simulink library "NeuroModelerLibrary"  (Simulink 10.2)
settings: Solver=ode45  StartTime=0.0  StopTime=10.0  RelTol=1e-3
libraries: $bdroot x672, simulink x5, neural x2
(part 2 of 5)

== system NeuroModelerLibrary/Neuron Elements/IaF Compartment ==
  Synapses : Inport
  Resting Potential : Inport  Port=2
  Reset Signal : Inport  Port=3
  Constant1 : Constant  Value=V_reset
  Constant10 : Constant  Value=tau_m
  Constant12 : Constant  Value=I_const
  Gain3 : Gain  Gain=tau_m/Cm
  Inertial Link With Reset1 : $bdroot/Support/Inertial Link With Reset  SystemSampleTime=-1  VariantActivationTime=update diagram  Latency=0  AutoFrameSizeCalculation=off
  Sum1 : Sum
  Sum3 : Sum
  Out1 : Outport
  wires:
  Reset Signal/1 -> Inertial Link With Reset1/4
  Gain3/1 -> Sum3/1  "Input"
  Constant1/1 -> Inertial Link With Reset1/3
  Inertial Link With Reset1/1 -> Out1/1
  Sum3/1 -> Inertial Link With Reset1/1  "Value"
  Constant12/1 -> Sum1/2
  Sum1/1 -> Gain3/1
  Synapses/1 -> Sum1/1
  Constant10/1 -> Inertial Link With Reset1/2
  Resting Potential/1 -> Sum3/2

== system NeuroModelerLibrary/Neuron Elements/IaF LTZone ==
  Potential : Inport
  Constant2 : Constant
  Constant6 : Constant  Value=0
  S1 : Switch  Threshold=V_th  SaturateOnIntegerOverflow=on  InputSameDT=on
  Out : Outport
  Out Potential : Outport  Port=2
  wires:
  S1/1 -> Out/1
  Potential/1 -> S1/2, Out Potential/1
  Constant6/1 -> S1/3
  Constant2/1 -> S1/1

== system NeuroModelerLibrary/Neuron Elements/Ion System ==
  Synapse : Inport
  Channel : Inport  Port=2
  Rm : Inport  Port=3
  Cm : Inport  Port=4
  Feedback : Inport  Port=5
  RFm : Inport  Port=6
  Divide : Product  Inputs=*/
  Divide1 : Product  Inputs=*/
  F1 : Fcn  Expr=-u
  F4 : Fcn  Expr=1/u
  Inertial Link : $bdroot/Support/Inertial Link  SystemSampleTime=-1  VariantActivationTime=update diagram  Latency=0  AutoFrameSizeCalculation=off
  P1 : Product  InputSameDT=on  RndMeth=Zero  SaturateOnIntegerOverflow=on  OutDataTypeStr=Inherit: Same as first input
  S2 : Switch  Criteria=u2 > Threshold  SaturateOnIntegerOverflow=on  InputSameDT=on
  Sum2 : Sum  InputSameDT=on  SaturateOnIntegerOverflow=on  OutDataTypeStr=Inherit: Same as first input
  Sum4 : Sum  Inputs=-+  InputSameDT=on  SaturateOnIntegerOverflow=on  OutDataTypeStr=Inherit: Same as first input
  Sum5 : Sum  InputSameDT=on  SaturateOnIntegerOverflow=on  OutDataTypeStr=Inherit: Same as first input
  Out : Outport  VectorParamsAs1DForOutWhenUnconnected=off
  wires:
  F1/1 -> Sum2/1
  Channel/1 -> Sum2/2
  Sum2/1 -> Sum4/2
  Feedback/1 -> F1/1, S2/2
  Rm/1 -> S2/3
  RFm/1 -> S2/1
  S2/1 -> F4/1
  Sum4/1 -> Inertial Link/1
  P1/1 -> Sum4/1
  Inertial Link/1 -> Out/1, P1/1
  Sum5/1 -> Divide/2
  Divide/1 -> Inertial Link/2
  Synapse/1 -> Divide1/1, Sum5/2
  F4/1 -> Divide1/2, Sum5/1
  Cm/1 -> Divide/1
  Divide1/1 -> P1/2

== system NeuroModelerLibrary/Neuron Elements/Ion System v0.1 ==
  Synapse : Inport
  Channel : Inport  Port=2
  Rm : Inport  Port=3
  Cm : Inport  Port=4
  Divide : Product  Inputs=**/  InputSameDT=on  RndMeth=Zero  OutDataTypeStr=Inherit: Same as first input
  F2 : Fcn  Expr=u
  F3 : Fcn  Expr=1/(1+abs(u))
  F4 : Fcn  Expr=1/u
  Inertial Link (H1) : Subsystem
  P1 : Product  InputSameDT=on  RndMeth=Zero  SaturateOnIntegerOverflow=on  OutDataTypeStr=Inherit: Same as first input
  Product : Product  InputSameDT=on  RndMeth=Zero  OutDataTypeStr=Inherit: Same as first input
  Sum1 : Sum  Inputs=-+  InputSameDT=on  SaturateOnIntegerOverflow=on  OutDataTypeStr=Inherit: Same as first input
  Sum4 : Sum  Inputs=-+  InputSameDT=on  SaturateOnIntegerOverflow=on  OutDataTypeStr=Inherit: Same as first input
  Sum5 : Sum  InputSameDT=on  SaturateOnIntegerOverflow=on  OutDataTypeStr=Inherit: Same as first input
  Out : Outport  VectorParamsAs1DForOutWhenUnconnected=off
  wires:
  Sum4/1 -> Inertial Link (H1)/1(In1)
  P1/1 -> Sum4/1
  Inertial Link (H1)/1(Out1) -> P1/1, Out/1, Sum1/2
  Sum5/1 -> Divide/3
  Divide/1 -> Inertial Link (H1)/2(In2)
  Synapse/1 -> Product/1, Sum5/2
  Channel/1 -> Sum4/2, Sum1/1
  Rm/1 -> F4/1, F2/1
  F4/1 -> Sum5/1
  Cm/1 -> Divide/1
  F2/1 -> Product/2
  Product/1 -> P1/2
  F3/1 -> Divide/2
  Sum1/1 -> F3/1

== system NeuroModelerLibrary/Neuron Elements/LTZone ==
  Potential : Inport
  E : Inport  Port=2
  C5 : Constant  Value=0
  FB : Gain  Gain=FB  OutDataTypeStr=Inherit: Same as input  ParamDataTypeStr=Inherit: Same as input
  Inputs : Gain  Gain=1/NM  OutDataTypeStr=Inherit: Same as input  ParamDataTypeStr=Inherit: Same as input
  Relay : Relay  OnSwitchValue=T  OffSwitchValue=0
  S2 : Switch  Threshold=1  SaturateOnIntegerOverflow=on  InputSameDT=on
  S3 : Switch  Threshold=1  SaturateOnIntegerOverflow=on  InputSameDT=on
  Transfer Fcn : TransferFcn  Denominator=[IT 1]
  Feedback : Outport  InitialOutput=0  VectorParamsAs1DForOutWhenUnconnected=off
  Visual : Outport  Port=2  InitialOutput=0  VectorParamsAs1DForOutWhenUnconnected=off
  Out : Outport  Port=3  InitialOutput=0  VectorParamsAs1DForOutWhenUnconnected=off
  wires:
  Transfer Fcn/1 -> S3/3, Relay/1
  S3/1 -> Visual/1
  Relay/1 -> S3/2, S2/2
  S2/1 -> FB/1, Out/1
  E/1 -> S2/1, S3/1
  C5/1 -> S2/3
  Potential/1 -> Inputs/1
  FB/1 -> Feedback/1
  Inputs/1 -> Transfer Fcn/1

== system NeuroModelerLibrary/Neuron Elements/LTZone v0.1 ==
  note: X1
  note: X2
  Sum : Inport
  E : Inport  Port=2
  C1 : Constant
  C2 : Constant  Value=1/Rc
  C3 : Constant  Value=1/RR
  C5 : Constant  Value=0
  F1 : Fcn  Expr=Cc/u
  Inertial Link (H1) : Subsystem
  Relay : Relay  OnSwitchValue=T  OffSwitchValue=0
  S1 : Switch  Threshold=1  SaturateOnIntegerOverflow=on  InputSameDT=on
  S2 : Switch  Threshold=1  SaturateOnIntegerOverflow=on  InputSameDT=on
  S3 : Switch  Threshold=1  SaturateOnIntegerOverflow=on  InputSameDT=on
  Sum2 : Sum  InputSameDT=on  SaturateOnIntegerOverflow=on  OutDataTypeStr=Inherit: Same as first input
  Transfer Fcn : TransferFcn  Denominator=[IT 1]
  Out : Outport  InitialOutput=0  VectorParamsAs1DForOutWhenUnconnected=off
  Membrane : Outport  Port=2  InitialOutput=0  VectorParamsAs1DForOutWhenUnconnected=off
  Visual : Outport  Port=3  InitialOutput=0  VectorParamsAs1DForOutWhenUnconnected=off
  wires:
  S3/1 -> Visual/1
  Relay/1 -> S3/2, S2/2, S1/2
  Transfer Fcn/1 -> Membrane/1, S3/3, Relay/1, Sum2/2
  S1/1 -> F1/1
  S2/1 -> Out/1, Sum2/1
  E/1 -> S3/1, S2/1
  C5/1 -> S2/3
  Sum/1 -> Transfer Fcn/1
  C3/1 -> S1/1
  C2/1 -> S1/3
  F1/1 -> Inertial Link (H1)/2(In2)
  Sum2/1 -> Inertial Link (H1)/1(In1)

== system NeuroModelerLibrary/Neuron Elements/LTZoneV2 ==
  Potential : Inport
  E : Inport  Port=2
  C1 : Constant  Value=inertia
  C5 : Constant  Value=0
  FB : Gain  Gain=FB  OutDataTypeStr=Inherit: Same as input  ParamDataTypeStr=Inherit: Same as input
  Inputs : Gain  Gain=1/NM  OutDataTypeStr=Inherit: Same as input  ParamDataTypeStr=Inherit: Same as input
  Relay : Relay  OnSwitchValue=T  OffSwitchValue=switchOff
  S2 : Switch  Threshold=1  SaturateOnIntegerOverflow=on  InputSameDT=on
  S3 : Switch  Threshold=1  SaturateOnIntegerOverflow=on  InputSameDT=on
  Switch : Switch  Threshold=1
  Transfer Fcn1 : TransferFcn  Denominator=[IT 1]
  Out : Outport  InitialOutput=0  VectorParamsAs1DForOutWhenUnconnected=off
  OutPotential : Outport  Port=2  InitialOutput=0  VectorParamsAs1DForOutWhenUnconnected=off
  Feedback : Outport  Port=3  InitialOutput=0  VectorParamsAs1DForOutWhenUnconnected=off
  Visual : Outport  Port=4  InitialOutput=0  VectorParamsAs1DForOutWhenUnconnected=off
  wires:
  Transfer Fcn1/1 -> Switch/1
  C1/1 -> Switch/2
  Inputs/1 -> Switch/3, Transfer Fcn1/1
  Switch/1 -> S3/3, OutPotential/1, Relay/1
  S3/1 -> Visual/1
  Relay/1 -> S3/2, S2/2
  S2/1 -> FB/1, Out/1
  E/1 -> S2/1, S3/1
  C5/1 -> S2/3
  Potential/1 -> Inputs/1
  FB/1 -> Feedback/1

== system NeuroModelerLibrary/Neuron Elements/Multistate Membrane ==
  Excitatory Synapse : Inport
  Excitatory input : Inport  Port=2
  Feedback : Inport  Port=3
  Arresting input : Inport  Port=4
  Arresting Synapse : Inport  Port=5
  Gain5 : Gain  Gain=0.5  OutDataTypeStr=Inherit: Same as input  ParamDataTypeStr=Inherit: Same as input
  Gain6 : Gain  Gain=0.5  OutDataTypeStr=Inherit: Same as input  ParamDataTypeStr=Inherit: Same as input
  Simple Membrane : $bdroot/Neuron Elements/Simple Membrane  ACm=1e-9  ARm=1e7  ECm=1e-9  ERm=1e7  ARFm=1e8  ERFm=1e8
  Simple Membrane1 : $bdroot/Neuron Elements/Simple Membrane  ACm=1e-9  ARm=1e7  ECm=1e-9  ERm=1e7  ARFm=1e8  ERFm=1e8
  Sum{1,3,8..11} (6 alike) : Sum  InputSameDT=on  SaturateOnIntegerOverflow=on  OutDataTypeStr=Inherit: Same as first input
  Out1 : Outport  VectorParamsAs1DForOutWhenUnconnected=off
  Out3 : Outport  Port=2  VectorParamsAs1DForOutWhenUnconnected=off
  wires:
  Arresting input/1 -> Sum9/1, Sum11/1
  Sum1/1 -> Gain5/1
  Sum3/1 -> Gain6/1
  Simple Membrane/2 -> Sum3/1, Sum11/2
  Simple Membrane/1 -> Sum1/1, Sum10/1
  Gain5/1 -> Out1/1
  Gain6/1 -> Out3/1
  Sum8/1 -> Simple Membrane/2
  Sum9/1 -> Simple Membrane/4
  Sum10/1 -> Simple Membrane1/2
  Sum11/1 -> Simple Membrane1/4
  Simple Membrane1/1 -> Sum9/2, Sum1/2
  Simple Membrane1/2 -> Sum8/1, Sum3/2
  Feedback/1 -> Simple Membrane/3, Simple Membrane1/3
  Excitatory Synapse/1 -> Simple Membrane1/1
  Arresting Synapse/1 -> Simple Membrane1/5
  Excitatory input/1 -> Sum8/2, Sum10/2

== system NeuroModelerLibrary/Neuron Elements/Neuro Membrane v0.1 ==
  Excitatory Synapse : Inport
  Excitatory Channel : Inport  Port=2
  Recharge : Inport  Port=3
  Arresting Channel : Inport  Port=4
  Arresting Synapse : Inport  Port=5
  ACm : Constant  Value=ACm
  ARm : Constant  Value=ARm
  ECm : Constant  Value=ECm
  ERm : Constant  Value=ERm
  Neuro Channel : $bdroot/Neuron Elements/Ion System v0.1  SystemSampleTime=-1  VariantActivationTime=update diagram  Latency=0  AutoFrameSizeCalculation=off
  Neuro Channel1 : $bdroot/Neuron Elements/Ion System v0.1  SystemSampleTime=-1  VariantActivationTime=update diagram  Latency=0  AutoFrameSizeCalculation=off
  Sum1 : Sum  Inputs=-+  InputSameDT=on  SaturateOnIntegerOverflow=on  OutDataTypeStr=Inherit: Same as first input
  Sum2 : Sum  Inputs=+-  InputSameDT=on  SaturateOnIntegerOverflow=on  OutDataTypeStr=Inherit: Same as first input
  Excitatory Out : Outport  VectorParamsAs1DForOutWhenUnconnected=off
  Arresting Out : Outport  Port=2  VectorParamsAs1DForOutWhenUnconnected=off
  wires:
  Recharge/1 -> Sum2/2, Sum1/1
  Arresting Channel/1 -> Sum2/1
  Sum2/1 -> Neuro Channel/2
  Sum1/1 -> Neuro Channel1/2
  Excitatory Channel/1 -> Sum1/2
  Arresting Synapse/1 -> Neuro Channel1/1
  Excitatory Synapse/1 -> Neuro Channel/1
  Neuro Channel/1 -> Arresting Out/1
  Neuro Channel1/1 -> Excitatory Out/1
  ERm/1 -> Neuro Channel1/3
  ECm/1 -> Neuro Channel1/4
  ARm/1 -> Neuro Channel/3
  ACm/1 -> Neuro Channel/4

== system NeuroModelerLibrary/Neuron Elements/Simple Membrane ==
  Excitatory Synapse : Inport
  Excitatory input : Inport  Port=2
  Feedback : Inport  Port=3
  Arresting input : Inport  Port=4
  Arresting Synapse : Inport  Port=5
  ACm : Constant  Value=ACm
  ARm : Constant  Value=ARm
  ARm1 : Constant  Value=ARFm
  ECm : Constant  Value=ECm
  ERm : Constant  Value=ERm
  ERm1 : Constant  Value=ERFm
  Ion System : $bdroot/Neuron Elements/Ion System
  Ion System1 : $bdroot/Neuron Elements/Ion System
  Excitatory Out : Outport  VectorParamsAs1DForOutWhenUnconnected=off
  Arresting Out : Outport  Port=2  VectorParamsAs1DForOutWhenUnconnected=off
  wires:
  Arresting input/1 -> Ion System/2
  Feedback/1 -> Ion System/5, Ion System1/5
  ARm1/1 -> Ion System/6
  Excitatory input/1 -> Ion System1/2
  Arresting Synapse/1 -> Ion System1/1
  Excitatory Synapse/1 -> Ion System/1
  ERm/1 -> Ion System1/3
  ECm/1 -> Ion System1/4
  ARm/1 -> Ion System/3
  ACm/1 -> Ion System/4
  Ion System/1 -> Arresting Out/1
  ERm1/1 -> Ion System1/6
  Ion System1/1 -> Excitatory Out/1

== system NeuroModelerLibrary/Neuron Elements/Synapse ==
  In1 : Inport
  Constant1 : Constant  Value=0
  Constant2 : Constant  Value=UseKsi
  Constant4 : Constant  Value=DecompositionTC
  Constant5 : Constant  Value=SecretionTC
  Fcn : Fcn  Expr=u*u*ksi
  Gain : Gain  Gain=4*ksi/gamma  SaturateOnIntegerOverflow=on  OutDataTypeStr=Inherit: Same as input  ParamDataTypeStr=Inherit: Same as input
  Gain1 : Gain  SaturateOnIntegerOverflow=on  OutDataTypeStr=Inherit: Same as input  ParamDataTypeStr=Inherit: Same as input
  Gain2 : Gain  Gain=1/gamma  SaturateOnIntegerOverflow=on  OutDataTypeStr=Inherit: Same as input  ParamDataTypeStr=Inherit: Same as input
  Inertial Link : $bdroot/Support/Inertial Link
  Sum : Sum  Inputs=+-  SaturateOnIntegerOverflow=on
  Switch1 : Switch
  Switch2 : Switch  Threshold=1
  Switch3 : Switch  Threshold=1
  Out1 : Outport  VectorParamsAs1DForOutWhenUnconnected=off
  wires:
  Fcn/1 -> Sum/2
  In1/1 -> Switch2/2, Gain1/1
  Sum/1 -> Gain/1
  Inertial Link/1 -> Gain2/1, Fcn/1, Sum/1
  Constant4/1 -> Switch2/3
  Constant5/1 -> Switch2/1
  Switch2/1 -> Inertial Link/2
  Constant1/1 -> Switch1/3
  Gain1/1 -> Inertial Link/1
  Switch1/1 -> Out1/1
  Gain/1 -> Switch3/1
  Switch3/1 -> Switch1/1, Switch1/2
  Constant2/1 -> Switch3/2
  Gain2/1 -> Switch3/3

== system NeuroModelerLibrary/Neuron Elements/Synapse Ion System v0.1 ==
  Synapse : Inport
  Channel : Inport  Port=2
  Rm : Inport  Port=3
  Cm : Inport  Port=4
  Divide : Product  Inputs=**/  InputSameDT=on  RndMeth=Zero  OutDataTypeStr=Inherit: Same as first input
  F2 : Fcn  Expr=u
  F3 : Fcn  Expr=1/(1+abs(u))
  F4 : Fcn  Expr=1/u
  Inertial Link (H1) : Subsystem
  P1 : Product  Inputs=3  InputSameDT=on  RndMeth=Zero  SaturateOnIntegerOverflow=on  OutDataTypeStr=Inherit: Same as first input
  Product : Product  InputSameDT=on  RndMeth=Zero  OutDataTypeStr=Inherit: Same as first input
  Sum1 : Sum  Inputs=-+  InputSameDT=on  SaturateOnIntegerOverflow=on  OutDataTypeStr=Inherit: Same as first input
  Sum4 : Sum  Inputs=-+  InputSameDT=on  SaturateOnIntegerOverflow=on  OutDataTypeStr=Inherit: Same as first input
  Sum5 : Sum  InputSameDT=on  SaturateOnIntegerOverflow=on  OutDataTypeStr=Inherit: Same as first input
  Out : Outport  VectorParamsAs1DForOutWhenUnconnected=off
  wires:
  Sum1/1 -> F3/1
  Product/1 -> P1/2
  F2/1 -> Product/2
  F4/1 -> Sum5/1
  Rm/1 -> F2/1, F4/1
  Channel/1 -> Sum1/1, Sum4/2
  Synapse/1 -> Sum5/2, Product/1, P1/3
  Divide/1 -> Inertial Link (H1)/2(In2)
  Sum5/1 -> Divide/3
  Inertial Link (H1)/1(Out1) -> Sum1/2, Out/1, P1/1
  P1/1 -> Sum4/1
  Sum4/1 -> Inertial Link (H1)/1(In1)
  F3/1 -> Divide/1
  Cm/1 -> Divide/2

== system NeuroModelerLibrary/Neuron Elements/Synapse Membrane v0.1 ==
  Excitatory Synapse : Inport
  Excitatory Channel : Inport  Port=2
  Recharge : Inport  Port=3
  Arresting Channel : Inport  Port=4
  Arresting Synapse : Inport  Port=5
  ACm : Constant  Value=ACm
  ARm : Constant  Value=ARm
  ECm : Constant  Value=ECm
  ERm : Constant  Value=ERm
  Sum1 : Sum  Inputs=-+  InputSameDT=on  SaturateOnIntegerOverflow=on  OutDataTypeStr=Inherit: Same as first input
  Sum2 : Sum  Inputs=+-  InputSameDT=on  SaturateOnIntegerOverflow=on  OutDataTypeStr=Inherit: Same as first input
  Synapse Channel : $bdroot/Neuron Elements/Synapse Ion System v0.1  SystemSampleTime=-1  VariantActivationTime=update diagram  Latency=0  AutoFrameSizeCalculation=off
  Synapse Channel1 : $bdroot/Neuron Elements/Synapse Ion System v0.1  SystemSampleTime=-1  VariantActivationTime=update diagram  Latency=0  AutoFrameSizeCalculation=off
  Excitatory Out : Outport  VectorParamsAs1DForOutWhenUnconnected=off
  Arresting Out : Outport  Port=2  VectorParamsAs1DForOutWhenUnconnected=off
  wires:
  ACm/1 -> Synapse Channel/4
  ARm/1 -> Synapse Channel/3
  ECm/1 -> Synapse Channel1/4
  ERm/1 -> Synapse Channel1/3
  Synapse Channel1/1 -> Excitatory Out/1
  Synapse Channel/1 -> Arresting Out/1
  Excitatory Synapse/1 -> Synapse Channel/1
  Arresting Synapse/1 -> Synapse Channel1/1
  Excitatory Channel/1 -> Sum1/2
  Sum1/1 -> Synapse Channel1/2
  Sum2/1 -> Synapse Channel/2
  Arresting Channel/1 -> Sum2/1
  Recharge/1 -> Sum1/1, Sum2/2

== system NeuroModelerLibrary/Neuron Elements/Synapse v0.1 ==
  In1 : Inport
  Constant1 : Constant  Value=0
  Constant4 : Constant  Value=DecompositionTC
  Constant5 : Constant  Value=SecretionTC
  Fcn : Fcn  Expr=u*u*ksi
  Fcn1 : Fcn  Expr=u/(u+ksi)
  Gain : Gain  Gain=gamma*4*ksi  SaturateOnIntegerOverflow=on  OutDataTypeStr=Inherit: Same as input  ParamDataTypeStr=Inherit: Same as input
  Gain1 : Gain  Gain=0.01  SaturateOnIntegerOverflow=on  OutDataTypeStr=Inherit: Same as input  ParamDataTypeStr=Inherit: Same as input
  Inertial Link (H1)1 : Subsystem
  Sum : Sum  Inputs=+-  InputSameDT=on  SaturateOnIntegerOverflow=on  OutDataTypeStr=Inherit: Same as first input
  Switch1 : Switch  SaturateOnIntegerOverflow=on  InputSameDT=on
  Switch2 : Switch  Threshold=1  SaturateOnIntegerOverflow=on  InputSameDT=on
  Out1 : Outport  VectorParamsAs1DForOutWhenUnconnected=off
  wires:
  Fcn/1 -> Sum/2
  In1/1 -> Switch2/2, Gain1/1
  Sum/1 -> Gain/1
  Inertial Link (H1)1/1(Out1) -> Fcn/1, Sum/1
  Constant4/1 -> Switch2/3
  Constant5/1 -> Switch2/1
  Switch2/1 -> Inertial Link (H1)1/2(In2)
  Gain/1 -> Switch1/2, Switch1/1
  Constant1/1 -> Switch1/3
  Gain1/1 -> Inertial Link (H1)1/1(In1)
  Switch1/1 -> Out1/1

== system NeuroModelerLibrary/Pacemaker Cells/Pacemaker1-1 Cell ==
  Stimulate1 : Inport
  Stimulate2 : Inport  Port=2
  Stimulate3 : Inport  Port=3
  Stimulate4 : Inport  Port=4
  Arresting1 : Inport  Port=5
  Arresting2 : Inport  Port=6
  Arresting3 : Inport  Port=7
  Arresting4 : Inport  Port=8
  C1 : Constant
  C2 : Constant
  C3 : Constant  Value=-0.99
  LTZone : $bdroot/Neuron Elements/LTZone  SystemSampleTime=-1  NM=1  FB=1.7  IT=0.005  T=0.001
  Simple Membrane{,1..3} (4 alike) : $bdroot/Neuron Elements/Simple Membrane  SystemSampleTime=-1  ACm=1e-9  ARm=1e7  ECm=1e-9  ERm=1e7  ARFm=1e8  ERFm=1e8
  Sum12 : Sum  InputSameDT=on  SaturateOnIntegerOverflow=on  OutDataTypeStr=Inherit: Same as first input
  Sum7 : Sum  InputSameDT=on  SaturateOnIntegerOverflow=on  OutDataTypeStr=Inherit: Same as first input
  Synapse{,1..7} (8 alike) : $bdroot/Neuron Elements/Synapse  SystemSampleTime=-1  SecretionTC=0.001  DecompositionTC=0.01  ksi=2  gamma=1e8
  Out : Outport  VectorParamsAs1DForOutWhenUnconnected=off
  Visual : Outport  Port=2  VectorParamsAs1DForOutWhenUnconnected=off
  Potential : Outport  Port=3  VectorParamsAs1DForOutWhenUnconnected=off
  wires:
  Synapse7/1 -> Simple Membrane/5
  Arresting4/1 -> Synapse7/1
  Synapse6/1 -> Simple Membrane1/5
  Arresting3/1 -> Synapse6/1
  Synapse5/1 -> Simple Membrane2/5
  Arresting2/1 -> Synapse5/1
  Stimulate4/1 -> Synapse/1
  Synapse/1 -> Simple Membrane/1
  Stimulate3/1 -> Synapse1/1
  Synapse1/1 -> Simple Membrane1/1
  Stimulate2/1 -> Synapse2/1
  Synapse2/1 -> Simple Membrane2/1
  Synapse3/1 -> Simple Membrane3/1
  C2/1 -> Simple Membrane3/2
  C3/1 -> Simple Membrane3/4
  Synapse4/1 -> Simple Membrane3/5
  Simple Membrane3/2 -> Simple Membrane2/4
  Simple Membrane3/1 -> Simple Membrane2/2
  Simple Membrane2/2 -> Simple Membrane1/4
  Simple Membrane2/1 -> Simple Membrane1/2
  LTZone/2 -> Visual/1
  LTZone/3 -> Out/1
  C1/1 -> LTZone/2
  Stimulate1/1 -> Synapse3/1
  Arresting1/1 -> Synapse4/1
  Simple Membrane1/1 -> Sum12/1, Simple Membrane/2
  Simple Membrane1/2 -> Sum12/2, Simple Membrane/4
  Sum7/1 -> Potential/1, LTZone/1
  LTZone/1 -> Simple Membrane/3
  Simple Membrane/1 -> Sum7/1
  Simple Membrane/2 -> Sum7/2

== system NeuroModelerLibrary/Pacemaker Cells/Pacemaker1-2 Cell ==
  Stimulate1 : Inport
  Stimulate2 : Inport  Port=2
  Stimulate3 : Inport  Port=3
  Stimulate4 : Inport  Port=4
  Arresting1 : Inport  Port=5
  Arresting2 : Inport  Port=6
  Arresting3 : Inport  Port=7
  Arresting4 : Inport  Port=8
  C1 : Constant
  C2 : Constant
  C3 : Constant  Value=-0.99
  LTZone : $bdroot/Neuron Elements/LTZone  NM=1  FB=1.7  IT=0.005  T=0.001
  Simple Membrane{,1..3} (4 alike) : $bdroot/Neuron Elements/Simple Membrane  ACm=1e-9  ARm=1e7  ECm=1e-9  ERm=1e7  ARFm=1e8  ERFm=1e8
  Sum12 : Sum  InputSameDT=on  SaturateOnIntegerOverflow=on  OutDataTypeStr=Inherit: Same as first input
  Sum7 : Sum  InputSameDT=on  SaturateOnIntegerOverflow=on  OutDataTypeStr=Inherit: Same as first input
  Synapse{,1..7} (8 alike) : $bdroot/Neuron Elements/Synapse  SecretionTC=0.001  DecompositionTC=0.01  UseKsi=on  ksi=2  gamma=1e8
  Out : Outport  VectorParamsAs1DForOutWhenUnconnected=off
  Visual : Outport  Port=2  VectorParamsAs1DForOutWhenUnconnected=off
  Potential : Outport  Port=3  VectorParamsAs1DForOutWhenUnconnected=off
  wires:
  Simple Membrane/2 -> Sum7/2
  Simple Membrane/1 -> Sum7/1
  LTZone/1 -> Simple Membrane/3, Simple Membrane1/3
  Sum7/1 -> LTZone/1, Potential/1
  Simple Membrane1/2 -> Simple Membrane/4, Sum12/2
  Simple Membrane1/1 -> Simple Membrane/2, Sum12/1
  Arresting1/1 -> Synapse4/1
  Stimulate1/1 -> Synapse3/1
  C1/1 -> LTZone/2
  LTZone/3 -> Out/1
  LTZone/2 -> Visual/1
  Simple Membrane2/1 -> Simple Membrane1/2
  Simple Membrane2/2 -> Simple Membrane1/4
  Simple Membrane3/1 -> Simple Membrane2/2
  Simple Membrane3/2 -> Simple Membrane2/4
  Synapse4/1 -> Simple Membrane3/5
  C3/1 -> Simple Membrane3/4
  C2/1 -> Simple Membrane3/2
  Synapse3/1 -> Simple Membrane3/1
  Synapse2/1 -> Simple Membrane2/1
  Stimulate2/1 -> Synapse2/1
  Synapse1/1 -> Simple Membrane1/1
  Stimulate3/1 -> Synapse1/1
  Synapse/1 -> Simple Membrane/1
  Stimulate4/1 -> Synapse/1
  Arresting2/1 -> Synapse5/1
  Synapse5/1 -> Simple Membrane2/5
  Arresting3/1 -> Synapse6/1
  Synapse6/1 -> Simple Membrane1/5
  Arresting4/1 -> Synapse7/1
  Synapse7/1 -> Simple Membrane/5

== system NeuroModelerLibrary/Pacemaker Cells/Pacemaker1-3 Cell ==
  Stimulate1 : Inport
  Stimulate2 : Inport  Port=2
  Stimulate3 : Inport  Port=3
  Stimulate4 : Inport  Port=4
  Arresting1 : Inport  Port=5
  Arresting2 : Inport  Port=6
  Arresting3 : Inport  Port=7
  Arresting4 : Inport  Port=8
  C1 : Constant
  C2 : Constant
  C3 : Constant  Value=-0.99
  LTZone : $bdroot/Neuron Elements/LTZone  SystemSampleTime=-1  NM=1  FB=1.7  IT=0.005  T=0.001
  Simple Membrane{,1..3} (4 alike) : $bdroot/Neuron Elements/Simple Membrane  SystemSampleTime=-1  ACm=1e-9  ARm=1e7  ECm=1e-9  ERm=1e7  ARFm=1e8  ERFm=1e8
  Sum12 : Sum  InputSameDT=on  SaturateOnIntegerOverflow=on  OutDataTypeStr=Inherit: Same as first input
  Sum7 : Sum  InputSameDT=on  SaturateOnIntegerOverflow=on  OutDataTypeStr=Inherit: Same as first input
  Synapse{,1..7} (8 alike) : $bdroot/Neuron Elements/Synapse  SystemSampleTime=-1  SecretionTC=0.001  DecompositionTC=0.01  ksi=2  gamma=1e8
  Out : Outport  VectorParamsAs1DForOutWhenUnconnected=off
  Visual : Outport  Port=2  VectorParamsAs1DForOutWhenUnconnected=off
  Potential : Outport  Port=3  VectorParamsAs1DForOutWhenUnconnected=off
  wires:
  Synapse7/1 -> Simple Membrane/5
  Arresting4/1 -> Synapse7/1
  Synapse6/1 -> Simple Membrane1/5
  Arresting3/1 -> Synapse6/1
  Synapse5/1 -> Simple Membrane2/5
  Arresting2/1 -> Synapse5/1
  Stimulate4/1 -> Synapse/1
  Synapse/1 -> Simple Membrane/1
  Stimulate3/1 -> Synapse1/1
  Synapse1/1 -> Simple Membrane1/1
  Stimulate2/1 -> Synapse2/1
  Synapse2/1 -> Simple Membrane2/1
  Synapse3/1 -> Simple Membrane3/1
  C2/1 -> Simple Membrane3/2
  C3/1 -> Simple Membrane3/4
  Synapse4/1 -> Simple Membrane3/5
  Simple Membrane3/2 -> Simple Membrane2/4
  Simple Membrane3/1 -> Simple Membrane2/2
  Simple Membrane2/2 -> Simple Membrane1/4
  Simple Membrane2/1 -> Simple Membrane1/2
  LTZone/2 -> Visual/1
  LTZone/3 -> Out/1
  C1/1 -> LTZone/2
  Stimulate1/1 -> Synapse3/1
  Arresting1/1 -> Synapse4/1
  Simple Membrane1/1 -> Sum12/1, Simple Membrane/2
  Simple Membrane1/2 -> Sum12/2, Simple Membrane/4
  Sum7/1 -> Potential/1, LTZone/1
  LTZone/1 -> Simple Membrane/3, Simple Membrane1/3, Simple Membrane2/3
  Simple Membrane/1 -> Sum7/1
  Simple Membrane/2 -> Sum7/2

== system NeuroModelerLibrary/Pacemaker Cells/Pacemaker1-4 Cell ==
  Stimulate1 : Inport
  Stimulate2 : Inport  Port=2
  Stimulate3 : Inport  Port=3
  Stimulate4 : Inport  Port=4
  Arresting1 : Inport  Port=5
  Arresting2 : Inport  Port=6
  Arresting3 : Inport  Port=7
  Arresting4 : Inport  Port=8
  C1 : Constant
  C2 : Constant
  C3 : Constant  Value=-0.99
  LTZone : $bdroot/Neuron Elements/LTZone  NM=1  FB=1.7  IT=0.005  T=0.001
  Simple Membrane{,1..3} (4 alike) : $bdroot/Neuron Elements/Simple Membrane  ACm=1e-9  ARm=1e7  ECm=1e-9  ERm=1e7  ARFm=1e8  ERFm=1e8
  Sum12 : Sum  InputSameDT=on  SaturateOnIntegerOverflow=on  OutDataTypeStr=Inherit: Same as first input
  Sum7 : Sum  InputSameDT=on  SaturateOnIntegerOverflow=on  OutDataTypeStr=Inherit: Same as first input
  Synapse{,1..7} (8 alike) : $bdroot/Neuron Elements/Synapse  SecretionTC=0.001  DecompositionTC=0.01  UseKsi=on  ksi=2  gamma=1e8
  Out : Outport  VectorParamsAs1DForOutWhenUnconnected=off
  Visual : Outport  Port=2  VectorParamsAs1DForOutWhenUnconnected=off
  Potential : Outport  Port=3  VectorParamsAs1DForOutWhenUnconnected=off
  wires:
  Synapse7/1 -> Simple Membrane/5
  Arresting4/1 -> Synapse7/1
  Synapse6/1 -> Simple Membrane1/5
  Arresting3/1 -> Synapse6/1
  Synapse5/1 -> Simple Membrane2/5
  Arresting2/1 -> Synapse5/1
  Stimulate4/1 -> Synapse/1
  Synapse/1 -> Simple Membrane/1
  Stimulate3/1 -> Synapse1/1
  Synapse1/1 -> Simple Membrane1/1
  Stimulate2/1 -> Synapse2/1
  Synapse2/1 -> Simple Membrane2/1
  Synapse3/1 -> Simple Membrane3/1
  C2/1 -> Simple Membrane3/2
  C3/1 -> Simple Membrane3/4
  Synapse4/1 -> Simple Membrane3/5
  Simple Membrane3/2 -> Simple Membrane2/4
  Simple Membrane3/1 -> Simple Membrane2/2
  Simple Membrane2/2 -> Simple Membrane1/4
  Simple Membrane2/1 -> Simple Membrane1/2
  LTZone/2 -> Visual/1
  LTZone/3 -> Out/1
  C1/1 -> LTZone/2
  Stimulate1/1 -> Synapse3/1
  Arresting1/1 -> Synapse4/1
  Simple Membrane1/1 -> Sum12/1, Simple Membrane/2
  Simple Membrane1/2 -> Sum12/2, Simple Membrane/4
  Sum7/1 -> Potential/1, LTZone/1
  LTZone/1 -> Simple Membrane/3, Simple Membrane1/3, Simple Membrane2/3, Simple Membrane3/3
  Simple Membrane/1 -> Sum7/1
  Simple Membrane/2 -> Sum7/2

== system NeuroModelerLibrary/Pacemaker Cells/Pacemaker2 Cell ==
  Stimulate1 : Inport
  Stimulate2 : Inport  Port=2
  Stimulate3 : Inport  Port=3
  Stimulate4 : Inport  Port=4
  Arresting1 : Inport  Port=5
  Arresting2 : Inport  Port=6
  Arresting3 : Inport  Port=7
  Arresting4 : Inport  Port=8
  C1 : Constant
  C2 : Constant
  C3 : Constant  Value=-0.99
  C4 : Constant
  C5 : Constant  Value=-1
  LTZone : $bdroot/Neuron Elements/LTZone  SystemSampleTime=-1  NM=2  FB=1.2  IT=0.005  T=0.001
  Simple Membrane{,1..4} (5 alike) : $bdroot/Neuron Elements/Simple Membrane  SystemSampleTime=-1  ACm=1e-9  ARm=1e7  ECm=1e-9  ERm=1e7  ARFm=1e8  ERFm=1e8
  Sum1 : Sum  InputSameDT=on  SaturateOnIntegerOverflow=on  OutDataTypeStr=Inherit: Same as first input
  Sum12 : Sum  InputSameDT=on  SaturateOnIntegerOverflow=on  OutDataTypeStr=Inherit: Same as first input
  Sum7 : Sum  Inputs=++++  InputSameDT=on  SaturateOnIntegerOverflow=on  OutDataTypeStr=Inherit: Same as first input
  Synapse{,1..7} (8 alike) : $bdroot/Neuron Elements/Synapse  SystemSampleTime=-1  SecretionTC=0.001  DecompositionTC=0.01  ksi=2  gamma=1e8
  Out : Outport  VectorParamsAs1DForOutWhenUnconnected=off
  Visual : Outport  Port=2  VectorParamsAs1DForOutWhenUnconnected=off
  Potential : Outport  Port=3  VectorParamsAs1DForOutWhenUnconnected=off
  wires:
  C5/1 -> Simple Membrane4/4
  C4/1 -> Simple Membrane4/2
  Simple Membrane/1 -> Sum7/2
  Simple Membrane/2 -> Sum7/3
  Simple Membrane4/2 -> Sum1/2
  Simple Membrane4/1 -> Sum1/1
  LTZone/1 -> Simple Membrane/3, Simple Membrane4/3
  Sum7/1 -> Potential/1, LTZone/1
  Simple Membrane1/2 -> Sum12/2, Simple Membrane/4
  Simple Membrane1/1 -> Sum12/1, Simple Membrane/2
  Arresting1/1 -> Synapse4/1
  Stimulate1/1 -> Synapse3/1
  C1/1 -> LTZone/2
  LTZone/3 -> Out/1
  LTZone/2 -> Visual/1
  Simple Membrane2/1 -> Simple Membrane1/2
  Simple Membrane2/2 -> Simple Membrane1/4
  Simple Membrane3/1 -> Simple Membrane2/2
  Simple Membrane3/2 -> Simple Membrane2/4
  Synapse4/1 -> Simple Membrane3/5
  C3/1 -> Simple Membrane3/4
  C2/1 -> Simple Membrane3/2
  Synapse3/1 -> Simple Membrane3/1
  Synapse2/1 -> Simple Membrane2/1
  Stimulate2/1 -> Synapse2/1
  Synapse1/1 -> Simple Membrane1/1
  Stimulate3/1 -> Synapse1/1
  Synapse/1 -> Simple Membrane/1
  Stimulate4/1 -> Synapse/1
  Arresting2/1 -> Synapse5/1
  Synapse5/1 -> Simple Membrane2/5
  Arresting3/1 -> Synapse6/1
  Synapse6/1 -> Simple Membrane1/5
  Arresting4/1 -> Synapse7/1
  Synapse7/1 -> Simple Membrane/5
  Sum1/1 -> Sum7/1

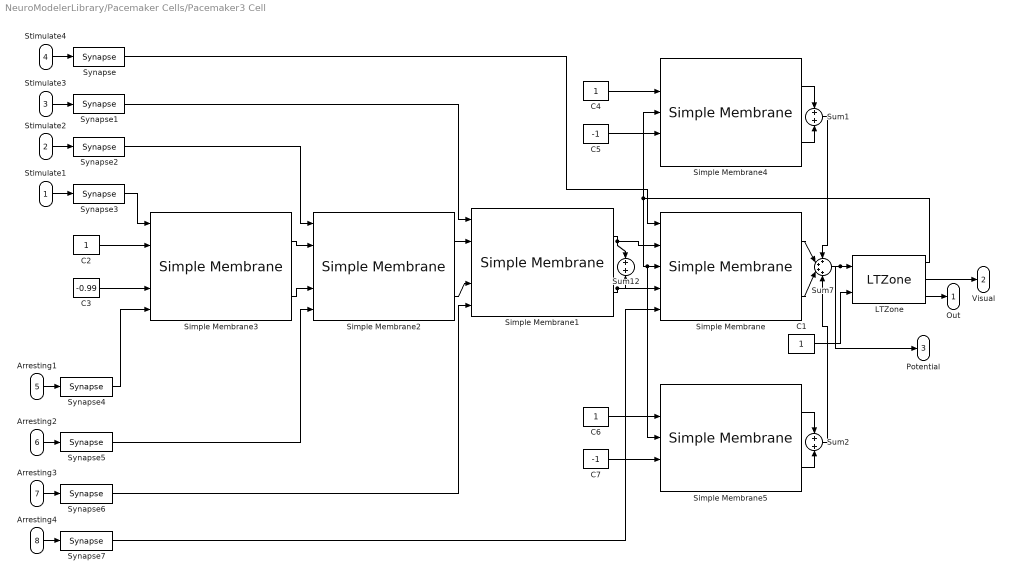
== system NeuroModelerLibrary/Pacemaker Cells/Pacemaker3 Cell ==
  Stimulate1 : Inport
  Stimulate2 : Inport  Port=2
  Stimulate3 : Inport  Port=3
  Stimulate4 : Inport  Port=4
  Arresting1 : Inport  Port=5
  Arresting2 : Inport  Port=6
  Arresting3 : Inport  Port=7
  Arresting4 : Inport  Port=8
  C{1..2,4,6} (4 alike) : Constant
  C3 : Constant  Value=-0.99
  C5 : Constant  Value=-1
  C7 : Constant  Value=-1
  LTZone : $bdroot/Neuron Elements/LTZone  SystemSampleTime=-1  NM=3  FB=1  IT=0.005  T=0.001
  Simple Membrane{,1..5} (6 alike) : $bdroot/Neuron Elements/Simple Membrane  SystemSampleTime=-1  ACm=1e-9  ARm=1e7  ECm=1e-9  ERm=1e7  ARFm=1e8  ERFm=1e8
  Sum1 : Sum  InputSameDT=on  SaturateOnIntegerOverflow=on  OutDataTypeStr=Inherit: Same as first input
  Sum12 : Sum  InputSameDT=on  SaturateOnIntegerOverflow=on  OutDataTypeStr=Inherit: Same as first input
  Sum2 : Sum  InputSameDT=on  SaturateOnIntegerOverflow=on  OutDataTypeStr=Inherit: Same as first input
  Sum7 : Sum  Inputs=++++  InputSameDT=on  SaturateOnIntegerOverflow=on  OutDataTypeStr=Inherit: Same as first input
  Synapse{,1..7} (8 alike) : $bdroot/Neuron Elements/Synapse  SystemSampleTime=-1  SecretionTC=0.001  DecompositionTC=0.01  ksi=2  gamma=1e8
  Out : Outport  VectorParamsAs1DForOutWhenUnconnected=off
  Visual : Outport  Port=2  VectorParamsAs1DForOutWhenUnconnected=off
  Potential : Outport  Port=3  VectorParamsAs1DForOutWhenUnconnected=off
  wires:
  Sum2/1 -> Sum7/4
  Simple Membrane5/1 -> Sum2/1
  Simple Membrane5/2 -> Sum2/2
  C6/1 -> Simple Membrane5/2
  C7/1 -> Simple Membrane5/4
  Synapse7/1 -> Simple Membrane/5
  Arresting4/1 -> Synapse7/1
  Synapse6/1 -> Simple Membrane1/5
  Arresting3/1 -> Synapse6/1
  Synapse5/1 -> Simple Membrane2/5
  Arresting2/1 -> Synapse5/1
  Stimulate4/1 -> Synapse/1
  Synapse/1 -> Simple Membrane/1
  Stimulate3/1 -> Synapse1/1
  Synapse1/1 -> Simple Membrane1/1
  Stimulate2/1 -> Synapse2/1
  Synapse2/1 -> Simple Membrane2/1
  Synapse3/1 -> Simple Membrane3/1
  C2/1 -> Simple Membrane3/2
  C3/1 -> Simple Membrane3/4
  Synapse4/1 -> Simple Membrane3/5
  Simple Membrane3/2 -> Simple Membrane2/4
  Simple Membrane3/1 -> Simple Membrane2/2
  Simple Membrane2/2 -> Simple Membrane1/4
  Simple Membrane2/1 -> Simple Membrane1/2
  LTZone/2 -> Visual/1
  LTZone/3 -> Out/1
  C1/1 -> LTZone/2
  Stimulate1/1 -> Synapse3/1
  Arresting1/1 -> Synapse4/1
  Simple Membrane1/1 -> Sum12/1, Simple Membrane/2
  Simple Membrane1/2 -> Sum12/2, Simple Membrane/4
  Sum7/1 -> Potential/1, LTZone/1
  LTZone/1 -> Simple Membrane/3, Simple Membrane5/3, Simple Membrane4/3
  Simple Membrane4/1 -> Sum1/1
  Simple Membrane4/2 -> Sum1/2
  Sum1/1 -> Sum7/1
  Simple Membrane/2 -> Sum7/3
  Simple Membrane/1 -> Sum7/2
  C4/1 -> Simple Membrane4/2
  C5/1 -> Simple Membrane4/4

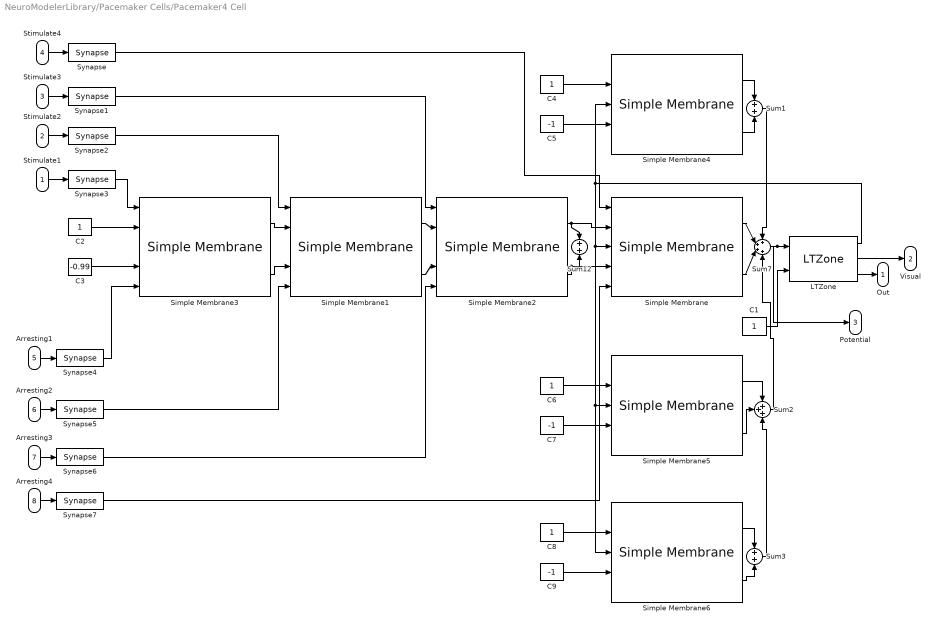
== system NeuroModelerLibrary/Pacemaker Cells/Pacemaker4 Cell ==
  Stimulate1 : Inport
  Stimulate2 : Inport  Port=2
  Stimulate3 : Inport  Port=3
  Stimulate4 : Inport  Port=4
  Arresting1 : Inport  Port=5
  Arresting2 : Inport  Port=6
  Arresting3 : Inport  Port=7
  Arresting4 : Inport  Port=8
  C{1..2,4,6,8} (5 alike) : Constant
  C3 : Constant  Value=-0.99
  C5 : Constant  Value=-1
  C7 : Constant  Value=-1
  C9 : Constant  Value=-1
  LTZone : $bdroot/Neuron Elements/LTZone  SystemSampleTime=-1  NM=4  FB=0.9  IT=0.005  T=0.001
  Simple Membrane{,1..6} (7 alike) : $bdroot/Neuron Elements/Simple Membrane  SystemSampleTime=-1  ACm=1e-9  ARm=1e7  ECm=1e-9  ERm=1e7  ARFm=1e8  ERFm=1e8
  Sum1 : Sum  InputSameDT=on  SaturateOnIntegerOverflow=on  OutDataTypeStr=Inherit: Same as first input
  Sum12 : Sum  InputSameDT=on  SaturateOnIntegerOverflow=on  OutDataTypeStr=Inherit: Same as first input
  Sum2 : Sum  Inputs=+++  InputSameDT=on  SaturateOnIntegerOverflow=on  OutDataTypeStr=Inherit: Same as first input
  Sum3 : Sum  InputSameDT=on  SaturateOnIntegerOverflow=on  OutDataTypeStr=Inherit: Same as first input
  Sum7 : Sum  Inputs=++++  InputSameDT=on  SaturateOnIntegerOverflow=on  OutDataTypeStr=Inherit: Same as first input
  Synapse{,1..7} (8 alike) : $bdroot/Neuron Elements/Synapse  SystemSampleTime=-1  SecretionTC=0.001  DecompositionTC=0.01  ksi=2  gamma=1e8
  Out : Outport  VectorParamsAs1DForOutWhenUnconnected=off
  Visual : Outport  Port=2  VectorParamsAs1DForOutWhenUnconnected=off
  Potential : Outport  Port=3  VectorParamsAs1DForOutWhenUnconnected=off
  wires:
  Sum3/1 -> Sum2/3
  Simple Membrane5/2 -> Sum2/2
  C9/1 -> Simple Membrane6/4
  C8/1 -> Simple Membrane6/2
  Simple Membrane6/2 -> Sum3/2
  Simple Membrane6/1 -> Sum3/1
  C5/1 -> Simple Membrane4/4
  C4/1 -> Simple Membrane4/2
  Simple Membrane/1 -> Sum7/2
  Simple Membrane/2 -> Sum7/3
  Sum1/1 -> Sum7/1
  Simple Membrane4/2 -> Sum1/2
  Simple Membrane4/1 -> Sum1/1
  LTZone/1 -> Simple Membrane5/3, Simple Membrane6/3, Simple Membrane/3, Simple Membrane4/3
  Sum7/1 -> Potential/1, LTZone/1
  Simple Membrane2/2 -> Sum12/2, Simple Membrane/4
  Simple Membrane2/1 -> Sum12/1, Simple Membrane/2
  Arresting1/1 -> Synapse4/1
  Stimulate1/1 -> Synapse3/1
  C1/1 -> LTZone/2
  LTZone/3 -> Out/1
  LTZone/2 -> Visual/1
  Simple Membrane1/1 -> Simple Membrane2/2
  Simple Membrane1/2 -> Simple Membrane2/4
  Simple Membrane3/1 -> Simple Membrane1/2
  Simple Membrane3/2 -> Simple Membrane1/4
  Synapse4/1 -> Simple Membrane3/5
  C3/1 -> Simple Membrane3/4
  C2/1 -> Simple Membrane3/2
  Synapse3/1 -> Simple Membrane3/1
  Synapse2/1 -> Simple Membrane1/1
  Stimulate2/1 -> Synapse2/1
  Synapse1/1 -> Simple Membrane2/1
  Stimulate3/1 -> Synapse1/1
  Synapse/1 -> Simple Membrane/1
  Stimulate4/1 -> Synapse/1
  Arresting2/1 -> Synapse5/1
  Synapse5/1 -> Simple Membrane1/5
  Arresting3/1 -> Synapse6/1
  Synapse6/1 -> Simple Membrane2/5
  Arresting4/1 -> Synapse7/1
  Synapse7/1 -> Simple Membrane/5
  C7/1 -> Simple Membrane5/4
  C6/1 -> Simple Membrane5/2
  Simple Membrane5/1 -> Sum2/1
  Sum2/1 -> Sum7/4

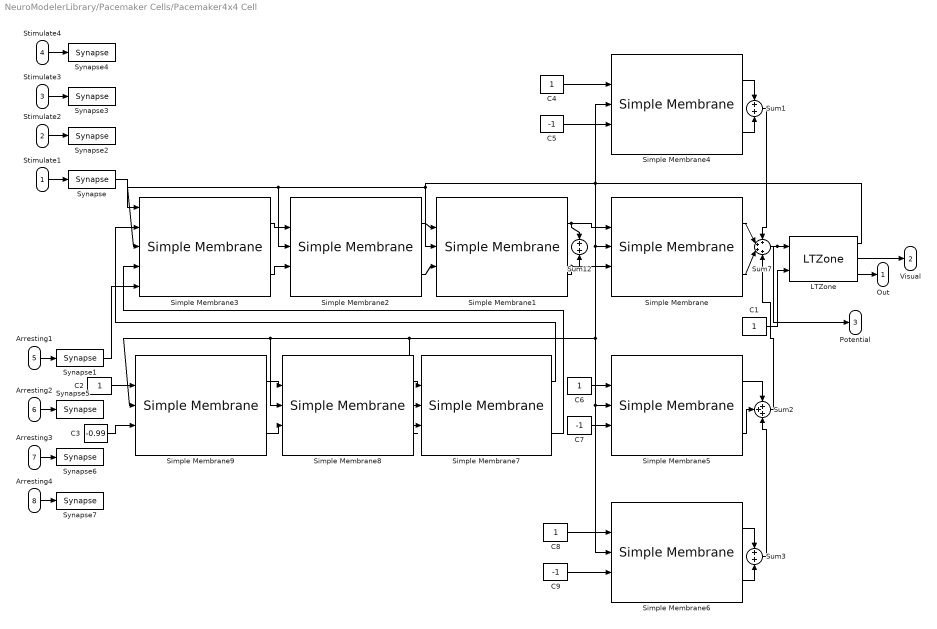
== system NeuroModelerLibrary/Pacemaker Cells/Pacemaker4x4 Cell ==
  Stimulate1 : Inport
  Stimulate2 : Inport  Port=2
  Stimulate3 : Inport  Port=3
  Stimulate4 : Inport  Port=4
  Arresting1 : Inport  Port=5
  Arresting2 : Inport  Port=6
  Arresting3 : Inport  Port=7
  Arresting4 : Inport  Port=8
  C{1..2,4,6,8} (5 alike) : Constant
  C3 : Constant  Value=-0.99
  C5 : Constant  Value=-1
  C7 : Constant  Value=-1
  C9 : Constant  Value=-1
  LTZone : $bdroot/LTZone  SystemSampleTime=-1  NM=4  FB=sqrt(4)  IT=0.005  T=0.001
  Simple Membrane{,1..9} (10 alike) : $bdroot/Simple Membrane  SystemSampleTime=-1  ACm=1e-9  ARm=1e7  ECm=1e-9  ERm=1e7  ARFm=1e8  ERFm=1e8
  Sum1 : Sum  InputSameDT=on  SaturateOnIntegerOverflow=on  OutDataTypeStr=Inherit: Same as first input
  Sum12 : Sum  InputSameDT=on  SaturateOnIntegerOverflow=on  OutDataTypeStr=Inherit: Same as first input
  Sum2 : Sum  Inputs=+++  InputSameDT=on  SaturateOnIntegerOverflow=on  OutDataTypeStr=Inherit: Same as first input
  Sum3 : Sum  InputSameDT=on  SaturateOnIntegerOverflow=on  OutDataTypeStr=Inherit: Same as first input
  Sum7 : Sum  Inputs=++++  InputSameDT=on  SaturateOnIntegerOverflow=on  OutDataTypeStr=Inherit: Same as first input
  Synapse{,1..7} (8 alike) : $bdroot/Synapse  SystemSampleTime=-1  SecretionTC=0.001  DecompositionTC=0.01  ksi=1  gamma=1e8
  Out : Outport  VectorParamsAs1DForOutWhenUnconnected=off
  Visual : Outport  Port=2  VectorParamsAs1DForOutWhenUnconnected=off
  Potential : Outport  Port=3  VectorParamsAs1DForOutWhenUnconnected=off
  wires:
  C3/1 -> Simple Membrane9/4
  C2/1 -> Simple Membrane9/2
  Simple Membrane9/2 -> Simple Membrane8/4
  Simple Membrane9/1 -> Simple Membrane8/2
  Simple Membrane8/2 -> Simple Membrane7/4
  Simple Membrane8/1 -> Simple Membrane7/2
  Simple Membrane7/1 -> Simple Membrane3/2
  Simple Membrane7/2 -> Simple Membrane3/4
  C9/1 -> Simple Membrane6/4
  C8/1 -> Simple Membrane6/2
  C7/1 -> Simple Membrane5/4
  C6/1 -> Simple Membrane5/2
  C5/1 -> Simple Membrane4/4
  C4/1 -> Simple Membrane4/2
  Sum3/1 -> Sum2/3
  Simple Membrane5/2 -> Sum2/2
  Simple Membrane6/2 -> Sum3/2
  Simple Membrane6/1 -> Sum3/1
  Simple Membrane/1 -> Sum7/2
  Simple Membrane/2 -> Sum7/3
  Sum1/1 -> Sum7/1
  Simple Membrane4/2 -> Sum1/2
  Simple Membrane4/1 -> Sum1/1
  LTZone/1 -> Simple Membrane3/3, Simple Membrane2/3, Simple Membrane1/3, Simple Membrane4/3, Simple Membrane9/3, Simple Membrane8/3, Simple Membrane7/3, Simple Membrane6/3, Simple Membrane5/3, Simple Membrane/3
  Sum7/1 -> LTZone/1, Potential/1
  Simple Membrane1/2 -> Simple Membrane/4, Sum12/2
  Simple Membrane1/1 -> Simple Membrane/2, Sum12/1
  Arresting1/1 -> Synapse1/1
  Stimulate1/1 -> Synapse/1
  C1/1 -> LTZone/2
  LTZone/3 -> Out/1
  LTZone/2 -> Visual/1
  Simple Membrane2/1 -> Simple Membrane1/2
  Simple Membrane2/2 -> Simple Membrane1/4
  Simple Membrane3/1 -> Simple Membrane2/2
  Simple Membrane3/2 -> Simple Membrane2/4
  Synapse1/1 -> Simple Membrane3/5
  Synapse/1 -> Simple Membrane3/1
  Stimulate2/1 -> Synapse2/1
  Stimulate3/1 -> Synapse3/1
  Stimulate4/1 -> Synapse4/1
  Arresting2/1 -> Synapse5/1
  Arresting3/1 -> Synapse6/1
  Arresting4/1 -> Synapse7/1
  Simple Membrane5/1 -> Sum2/1
  Sum2/1 -> Sum7/4

== system NeuroModelerLibrary/Pacemaker Cells/Slow Pacemaker Cell ==
  Stimulate1 : Inport
  Stimulate2 : Inport  Port=2
  Stimulate3 : Inport  Port=3
  Stimulate4 : Inport  Port=4
  Arresting1 : Inport  Port=5
  Arresting2 : Inport  Port=6
  Arresting3 : Inport  Port=7
  Arresting4 : Inport  Port=8
  C1 : Constant
  C2 : Constant
  C3 : Constant  Value=-0.99
  LTZone : $bdroot/Neuron Elements/LTZone  SystemSampleTime=-1  NM=1  FB=1.7  IT=0.005  T=0.001
  Simple Membrane : $bdroot/Neuron Elements/Simple Membrane  SystemSampleTime=-1  ACm=1e-9  ARm=1e8  ECm=1e-9  ERm=1e8  ARFm=1e8  ERFm=1e8
  Simple Membrane1 : $bdroot/Neuron Elements/Simple Membrane  SystemSampleTime=-1  ACm=1e-9  ARm=1e7  ECm=1e-9  ERm=1e7  ARFm=1e8  ERFm=1e8
  Simple Membrane2 : $bdroot/Neuron Elements/Simple Membrane  SystemSampleTime=-1  ACm=1e-9  ARm=1e7  ECm=1e-9  ERm=1e7  ARFm=1e8  ERFm=1e8
  Simple Membrane3 : $bdroot/Neuron Elements/Simple Membrane  SystemSampleTime=-1  ACm=1e-9  ARm=1e7  ECm=1e-9  ERm=1e7  ARFm=1e8  ERFm=1e8
  Sum12 : Sum  InputSameDT=on  SaturateOnIntegerOverflow=on  OutDataTypeStr=Inherit: Same as first input
  Sum7 : Sum  InputSameDT=on  SaturateOnIntegerOverflow=on  OutDataTypeStr=Inherit: Same as first input
  Synapse{,1..7} (8 alike) : $bdroot/Neuron Elements/Synapse  SystemSampleTime=-1  SecretionTC=0.001  DecompositionTC=0.01  ksi=2  gamma=1e8
  Out : Outport  VectorParamsAs1DForOutWhenUnconnected=off
  Visual : Outport  Port=2  VectorParamsAs1DForOutWhenUnconnected=off
  Potential : Outport  Port=3  VectorParamsAs1DForOutWhenUnconnected=off
  wires:
  Simple Membrane/2 -> Sum7/2
  Simple Membrane/1 -> Sum7/1
  LTZone/1 -> Simple Membrane/3
  Sum7/1 -> Potential/1, LTZone/1
  Simple Membrane1/2 -> Sum12/2, Simple Membrane/4
  Simple Membrane1/1 -> Sum12/1, Simple Membrane/2
  Arresting1/1 -> Synapse4/1
  Stimulate1/1 -> Synapse3/1
  C1/1 -> LTZone/2
  LTZone/3 -> Out/1
  LTZone/2 -> Visual/1
  Simple Membrane2/1 -> Simple Membrane1/2
  Simple Membrane2/2 -> Simple Membrane1/4
  Simple Membrane3/1 -> Simple Membrane2/2
  Simple Membrane3/2 -> Simple Membrane2/4
  Synapse4/1 -> Simple Membrane3/5
  C3/1 -> Simple Membrane3/4
  C2/1 -> Simple Membrane3/2
  Synapse3/1 -> Simple Membrane3/1
  Synapse2/1 -> Simple Membrane2/1
  Stimulate2/1 -> Synapse2/1
  Synapse1/1 -> Simple Membrane1/1
  Stimulate3/1 -> Synapse1/1
  Synapse/1 -> Simple Membrane/1
  Stimulate4/1 -> Synapse/1
  Arresting2/1 -> Synapse5/1
  Synapse5/1 -> Simple Membrane2/5
  Arresting3/1 -> Synapse6/1
  Synapse6/1 -> Simple Membrane1/5
  Arresting4/1 -> Synapse7/1
  Synapse7/1 -> Simple Membrane/5

== system NeuroModelerLibrary/Recycle Bin/Dendrite Neuron  Samples ==

== system NeuroModelerLibrary/Recycle Bin/Membrane Samples ==

== system NeuroModelerLibrary/Recycle Bin/Multistate Neuron  Samples ==

== system NeuroModelerLibrary/Recycle Bin/PCN1 ==

== system NeuroModelerLibrary/Recycle Bin/PCN2 ==

== system NeuroModelerLibrary/Recycle Bin/Pacemaker Samples ==

== system NeuroModelerLibrary/Recycle Bin/RCN ==

== system NeuroModelerLibrary/Recycle Bin/Simple  Neural Networks ==

== system NeuroModelerLibrary/Recycle Bin/Simple Neuron Samples ==

== system NeuroModelerLibrary/Recycle Bin/Size Neuron  Samples ==

== system NeuroModelerLibrary/Recycle Bin/Synapse Samples ==

== system NeuroModelerLibrary/Recycle Bin/TCN ==

== system NeuroModelerLibrary/Simple Cells/Afferent1 ==
  Stimulate : Inport
  C1 : Constant
  C2 : Constant  Value=0
  C3 : Constant  Value=-1
  Fcn : Fcn  Expr=2-exp(-ExpCoeff*(u+IncCoeff))
  LTZone : $bdroot/Neuron Elements/LTZone  NM=1  FB=1.7  IT=0.005  T=0.001
  Simple Membrane1 : $bdroot/Neuron Elements/Simple Membrane  ACm=1e-9  ARm=1e7  ECm=1e-9  ERm=1e7  ARFm=1e8  ERFm=1e8
  Sum1 : Sum  InputSameDT=on  SaturateOnIntegerOverflow=on  OutDataTypeStr=Inherit: Same as first input
  Sum7 : Sum  InputSameDT=on  SaturateOnIntegerOverflow=on  OutDataTypeStr=Inherit: Same as first input
  Out : Outport  VectorParamsAs1DForOutWhenUnconnected=off
  Visual : Outport  Port=2  VectorParamsAs1DForOutWhenUnconnected=off
  Potential : Outport  Port=3  VectorParamsAs1DForOutWhenUnconnected=off
  wires:
  Fcn/1 -> Sum1/1
  Sum1/1 -> Simple Membrane1/2
  Stimulate/1 -> Fcn/1
  C2/1 -> Sum1/2
  LTZone/1 -> Simple Membrane1/3
  Simple Membrane1/2 -> Sum7/2
  Simple Membrane1/1 -> Sum7/1
  LTZone/2 -> Visual/1
  LTZone/3 -> Out/1
  C1/1 -> LTZone/2
  Sum7/1 -> Potential/1, LTZone/1
  C3/1 -> Simple Membrane1/4

== system NeuroModelerLibrary/Simple Cells/Electric Simple Cell ==
  Chem Stimulate : Inport
  Chem Arresting : Inport  Port=2
  El Stimulate : Inport  Port=3
  El Arresting : Inport  Port=4
  C1 : Constant
  C2 : Constant
  C3 : Constant  Value=-1
  Inputs : Gain  Gain=0.5  OutDataTypeStr=Inherit: Same as input  ParamDataTypeStr=Inherit: Same as input
  Inputs1 : Gain  Gain=0.5  OutDataTypeStr=Inherit: Same as input  ParamDataTypeStr=Inherit: Same as input
  LTZone : $bdroot/Neuron Elements/LTZone  NM=1  FB=1.7  IT=0.005  T=0.001
  Simple Membrane : $bdroot/Neuron Elements/Simple Membrane  ACm=1e-9  ARm=1e7  ECm=1e-9  ERm=1e7  ARFm=1e8  ERFm=1e8
  Sum1 : Sum  InputSameDT=on  SaturateOnIntegerOverflow=on  OutDataTypeStr=Inherit: Same as first input
  Sum2 : Sum  InputSameDT=on  SaturateOnIntegerOverflow=on  OutDataTypeStr=Inherit: Same as first input
  Sum7 : Sum  InputSameDT=on  SaturateOnIntegerOverflow=on  OutDataTypeStr=Inherit: Same as first input
  Synapse : $bdroot/Neuron Elements/Synapse  SecretionTC=0.001  DecompositionTC=0.01  ksi=2  gamma=1e8
  Synapse1 : $bdroot/Neuron Elements/Synapse  SecretionTC=0.001  DecompositionTC=0.01  ksi=2  gamma=1e8
  Out : Outport  VectorParamsAs1DForOutWhenUnconnected=off
  Visual : Outport  Port=2  VectorParamsAs1DForOutWhenUnconnected=off
  Potential : Outport  Port=3  VectorParamsAs1DForOutWhenUnconnected=off
  Ex Potential : Outport  Port=4  VectorParamsAs1DForOutWhenUnconnected=off
  Ar Potential : Outport  Port=5  VectorParamsAs1DForOutWhenUnconnected=off
  wires:
  Synapse1/1 -> Simple Membrane/5
  Synapse/1 -> Simple Membrane/1
  Simple Membrane/2 -> Sum7/2, Ar Potential/1
  Simple Membrane/1 -> Sum7/1, Ex Potential/1
  LTZone/1 -> Simple Membrane/3
  Sum7/1 -> Potential/1, LTZone/1
  Chem Arresting/1 -> Synapse1/1
  Chem Stimulate/1 -> Synapse/1
  C1/1 -> LTZone/2
  LTZone/3 -> Out/1
  LTZone/2 -> Visual/1
  Sum1/1 -> Inputs/1
  Sum2/1 -> Inputs1/1
  C3/1 -> Sum2/2
  C2/1 -> Sum1/1
  El Stimulate/1 -> Sum1/2
  El Arresting/1 -> Sum2/1
  Inputs/1 -> Simple Membrane/2
  Inputs1/1 -> Simple Membrane/4

== system NeuroModelerLibrary/Simple Cells/Electric Simple2 Cell ==
  Chem Stimulate : Inport
  Chem Arresting : Inport  Port=2
  El Stimulate : Inport  Port=3
  El Arresting : Inport  Port=4
  C1 : Constant
  C2 : Constant
  C3 : Constant  Value=-1
  Inputs : Gain  Gain=0.5  OutDataTypeStr=Inherit: Same as input  ParamDataTypeStr=Inherit: Same as input
  Inputs1 : Gain  Gain=0.5  OutDataTypeStr=Inherit: Same as input  ParamDataTypeStr=Inherit: Same as input
  LTZone : $bdroot/Neuron Elements/LTZone  NM=1  FB=1.7  IT=0.005  T=0.001
  Simple Membrane : $bdroot/Neuron Elements/Simple Membrane  ACm=1e-9  ARm=1e7  ECm=1e-9  ERm=1e7  ARFm=1e8  ERFm=1e8
  Simple Membrane1 : $bdroot/Neuron Elements/Simple Membrane  ACm=1e-9  ARm=1e7  ECm=1e-9  ERm=1e7  ARFm=1e8  ERFm=1e8
  Sum1 : Sum  InputSameDT=on  SaturateOnIntegerOverflow=on  OutDataTypeStr=Inherit: Same as first input
  Sum2 : Sum  InputSameDT=on  SaturateOnIntegerOverflow=on  OutDataTypeStr=Inherit: Same as first input
  Sum7 : Sum  InputSameDT=on  SaturateOnIntegerOverflow=on  OutDataTypeStr=Inherit: Same as first input
  Synapse : $bdroot/Neuron Elements/Synapse  SecretionTC=0.001  DecompositionTC=0.01  UseKsi=on  ksi=2  gamma=1e8
  Synapse1 : $bdroot/Neuron Elements/Synapse  SecretionTC=0.001  DecompositionTC=0.01  UseKsi=on  ksi=2  gamma=1e8
  Out : Outport  VectorParamsAs1DForOutWhenUnconnected=off
  Visual : Outport  Port=2  VectorParamsAs1DForOutWhenUnconnected=off
  Potential : Outport  Port=3  VectorParamsAs1DForOutWhenUnconnected=off
  Ex Potential : Outport  Port=4  VectorParamsAs1DForOutWhenUnconnected=off
  Ar Potential : Outport  Port=5  VectorParamsAs1DForOutWhenUnconnected=off
  wires:
  El Arresting/1 -> Sum2/1
  El Stimulate/1 -> Sum1/2
  C2/1 -> Sum1/1
  C3/1 -> Sum2/2
  Sum2/1 -> Inputs1/1
  Sum1/1 -> Inputs/1
  LTZone/2 -> Visual/1
  LTZone/3 -> Out/1
  C1/1 -> LTZone/2
  Chem Stimulate/1 -> Synapse/1
  Chem Arresting/1 -> Synapse1/1
  Sum7/1 -> LTZone/1, Potential/1
  LTZone/1 -> Simple Membrane/3
  Simple Membrane/1 -> Sum7/1
  Simple Membrane/2 -> Sum7/2
  Inputs/1 -> Simple Membrane1/2
  Inputs1/1 -> Simple Membrane1/4
  Simple Membrane1/1 -> Simple Membrane/2, Ex Potential/1
  Simple Membrane1/2 -> Simple Membrane/4, Ar Potential/1
  Synapse/1 -> Simple Membrane1/1
  Synapse1/1 -> Simple Membrane1/5

== system NeuroModelerLibrary/Simple Cells/Large  NewNeuron v0.1 ==
  In1 : Inport
  In2 : Inport  Port=2
  In3 : Inport  Port=3
  In4 : Inport  Port=4
  In5 : Inport  Port=5
  C1 : Constant  Value=100
  C2 : Constant  Value=100
  Gain1 : Gain  Gain=0.5  OutDataTypeStr=Inherit: Same as input  ParamDataTypeStr=Inherit: Same as input
  Gain2 : Gain  Gain=-1  OutDataTypeStr=Inherit: Same as input  ParamDataTypeStr=Inherit: Same as input
  Gain3 : Gain  Gain=0.5  OutDataTypeStr=Inherit: Same as input  ParamDataTypeStr=Inherit: Same as input
  Gain4 : Gain  Gain=0.5  OutDataTypeStr=Inherit: Same as input  ParamDataTypeStr=Inherit: Same as input
  LTZone v0.1 : $bdroot/Neuron Elements/LTZone v0.1  Rc=1  Cc=0.001  RR=1  IT=0.005  T=10
  Neuro Membrane{,1..5} (6 alike) : $bdroot/Neuron Elements/Neuro Membrane v0.1  ACm=0.1  ARm=1  ECm=0.1  ERm=1
  Sum2 : Sum  InputSameDT=on  SaturateOnIntegerOverflow=on  OutDataTypeStr=Inherit: Same as first input
  Sum3 : Sum  InputSameDT=on  SaturateOnIntegerOverflow=on  OutDataTypeStr=Inherit: Same as first input
  Sum7 : Sum  Inputs=++++  InputSameDT=on  SaturateOnIntegerOverflow=on  OutDataTypeStr=Inherit: Same as first input
  Synapse{1..5} (5 alike) : $bdroot/Neuron Elements/Synapse v0.1  SecretionTC=0.001  DecompositionTC=0.1  ksi=1  gamma=1
  Out1 : Outport  VectorParamsAs1DForOutWhenUnconnected=off
  Out2 : Outport  Port=2  VectorParamsAs1DForOutWhenUnconnected=off
  Out3 : Outport  Port=3  VectorParamsAs1DForOutWhenUnconnected=off
  wires:
  Neuro Membrane4/2 -> Sum7/4
  Neuro Membrane4/1 -> Sum7/3
  Gain4/1 -> Neuro Membrane3/2
  Gain3/1 -> Neuro Membrane3/4
  LTZone v0.1/3 -> Out1/1
  Gain1/1 -> LTZone v0.1/1
  Neuro Membrane5/2 -> Sum3/2
  Neuro Membrane5/1 -> Sum2/2
  Sum2/1 -> Gain4/1
  Sum3/1 -> Gain3/1
  Neuro Membrane/2 -> Sum3/1
  Neuro Membrane/1 -> Sum2/1
  Neuro Membrane3/2 -> Neuro Membrane2/4
  Neuro Membrane3/1 -> Neuro Membrane2/2
  Neuro Membrane1/2 -> Neuro Membrane/4
  Neuro Membrane1/1 -> Neuro Membrane/2
  LTZone v0.1/1 -> Neuro Membrane2/3, Out2/1, Neuro Membrane4/3
  Synapse1/1 -> Neuro Membrane1/1
  In1/1 -> Synapse1/1
  C1/1 -> LTZone v0.1/2
  Neuro Membrane2/1 -> Sum7/1
  Sum7/1 -> Gain1/1
  Neuro Membrane2/2 -> Sum7/2
  Gain2/1 -> Neuro Membrane5/4, Neuro Membrane4/4, Neuro Membrane1/4
  C2/1 -> Gain2/1, Neuro Membrane5/2, Neuro Membrane4/2, Neuro Membrane1/2
  In2/1 -> Synapse2/1
  Synapse2/1 -> Neuro Membrane/1
  Synapse3/1 -> Neuro Membrane3/1
  In3/1 -> Synapse3/1
  Synapse4/1 -> Neuro Membrane2/1
  In4/1 -> Synapse4/1
  Synapse5/1 -> Neuro Membrane5/1
  In5/1 -> Synapse5/1
  LTZone v0.1/2 -> Out3/1
